simulink model "TrayectoriaVW_ACT"  (R2023b)
settings: Solver=VariableStepAuto  StartTime=0.0  StopTime=10.0  RelTol=1e-3
model workspace (MAT data in the model file):
  d = 0.21
libraries: SignalEditorBlockLib x1
settings Model: Creator=Alberto  LastModifiedBy=Alberto

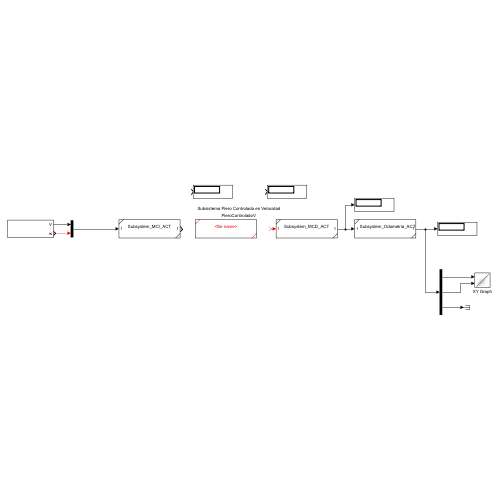
[thumbnail: Simulink's stored preview of the top-level diagram]
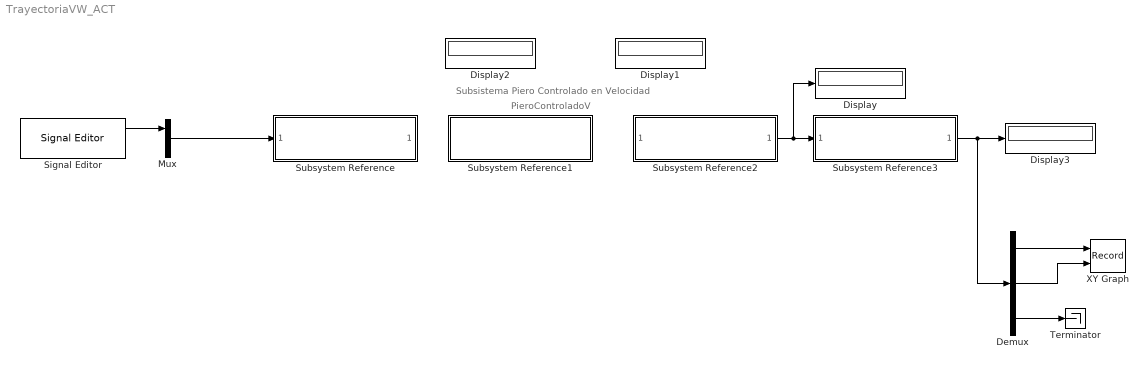
== system TrayectoriaVW_ACT ==
  note: PieroControladoV
  note: Subsistema Piero Controlado en Velocidad
  Demux : Demux  Outputs=3
  Display{,1..3} (4 alike) : Display
  Mux : Mux  Inputs=2
  Signal Editor : SignalEditorBlockLib/Signal Editor  FileName=C:\Users\Alberto\MATLAB\Projects\LabRob2024_SeguimientoIndividual\Data_ACT\SalirClase.mat  ActiveScenario=SalirClase  ActiveSignal=V  IsBus=off  OutputBusObjectStr=Bus: BusObject  SampleTime=0.01  Interpolate=off  ZeroCross=off  OutputAfterFinalValue=Setting to zero  Unit=inherit  PreserveSignalName=on  ApplySigPropsToAllScenarios=on  ApplySigPropsToAllSignals=on
  Subsystem Reference : Subsystem  ReferencedSubsystem=Subsystem_MCI_ACT
  Subsystem Reference1 : Subsystem  ReferencedSubsystem=<file name>
  Subsystem Reference2 : Subsystem  ReferencedSubsystem=Subsystem_MCD_ACT
  Subsystem Reference3 : Subsystem  ReferencedSubsystem=Subsystem_Odometria_ACT
  Terminator : Terminator
  XY Graph : Record  FileSettingsInternal="{\"entries\":[{\"content\":{\"excelSettings\":{\"content\":{},\"type\":\"Streamout.ExcelSettings\"}},\"type\":\"Streamout.FileSettingStorage\",\"uuid\":\"\"}],\"packageUris\":[\"http:\\/\\/schema.mathworks.com\\/mf0\\/streamout_blocks\\/R2020a\"],\"version\":\"1.0\"}"  Layout=[1 1]  SignalsInternal="{\"entries\":[{\"content\":{},\"type\":\"RecordBlkView.InputSignals\",\"uuid\":\"\"}],\"packageUris\":[\"http:\\/\\/schema.mathworks.com\\/mf0\\/streamout_blocks\\/R2020a\"],\"version\":\"1.0\"}"  VisualizationBindings="{\"xyplotplugin\":{\"info\":[{\"series\":[],\"subplotID\":1}]}}"  CompatibilityTag=XY
  wires:
  Subsystem Reference2/1 -> Display/1, Subsystem Reference3/1
  ? -> Subsystem Reference2/1
  Subsystem Reference3/1 -> Demux/1, Display3/1
  Demux/1 -> XY Graph/1
  Demux/2 -> XY Graph/2
  Demux/3 -> Terminator/1
  Signal Editor/1 -> Mux/1
  ? -> Mux/2
  Mux/1 -> Subsystem Reference/1

== system TrayectoriaVW_ACT/Subsystem Reference1 ==
